simulink model "FOSM"  (R2022b)
settings: Solver=VariableStepAuto  StartTime=0.0  StopTime=10.0  RelTol=1e-3
libraries: fod x2
settings Model: Creator=张倬境  LastModifiedBy=张倬境

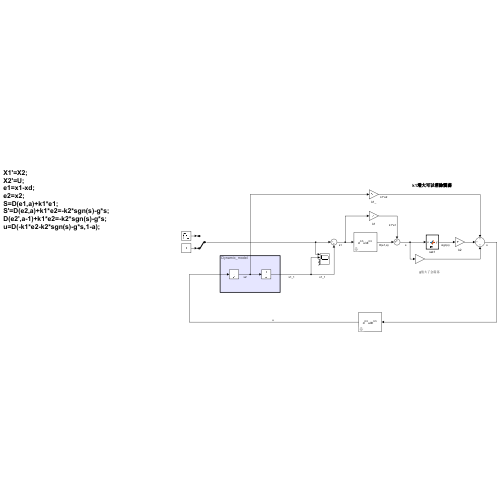
[thumbnail: Simulink's stored preview of the top-level diagram]
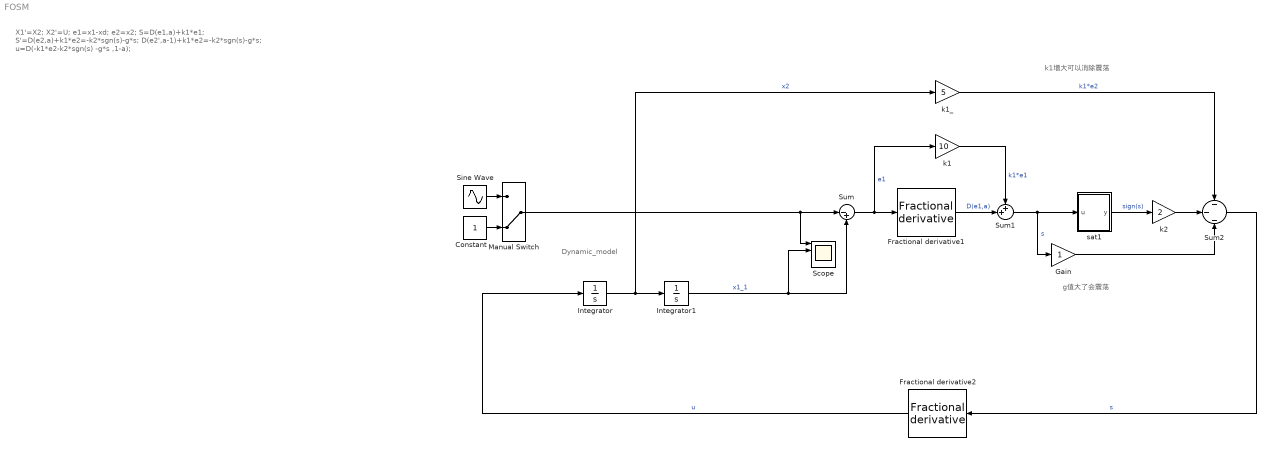
== system FOSM ==
  note: X1'=X2;
      | X2'=U;
      | e1=x1-xd;
      | e2=x2;
      | S=D(e1,a)+k1*e1;
      | S'=D(e2,a)+k1*e2=-k2*sgn(s)-g*s;
      | D(e2',a-1)+k1*e2=-k2*sgn(s)-g*s;
      | u=D(-k1*e2-k2*sgn(s) -g*s ,1-a);
  note: k1增大可以消除震荡
  note: Dynamic_model
  note: g值大了会震荡
  Constant : Constant
  Fractional derivative1 : fod/Fractional derivative  gam=0.5  ww=[0.001; 1000]  n=5  nFod=off
      settings: SourceProductName=FOMCON Toolbox
  Fractional derivative2 : fod/Fractional derivative  gam=0.5  ww=[0.001; 1000]  n=5  nFod=off
      settings: SourceProductName=FOMCON Toolbox
  Gain : Gain
  Integrator : Integrator
  Integrator1 : Integrator
  Manual Switch : ManualSwitch  CurrentSetting=0
  Scope : Scope  NumInputPorts=4
  Sine Wave : Sin  SampleTime=0
  Sum : Sum  Inputs=|-+
  Sum1 : Sum  Inputs=++|
  Sum2 : Sum  Inputs=-|-|-
  k1 : Gain  Gain=10
  k1_ : Gain  Gain=5
  k2 : Gain  Gain=2
  sat1 : MATLAB Function  TreatAsAtomicUnit=on
  wires:
  Sum/1 -> k1/1, Fractional derivative1/1  "e1"
  sat1/1(y) -> k2/1  "sign(s)"
  Gain/1 -> Sum2/3
  Integrator1/1 -> Scope/2, Sum/2  "x1_1"
  Manual Switch/1 -> Scope/1, Sum/1
  k2/1 -> Sum2/2
  Constant/1 -> Manual Switch/2
  k1/1 -> Sum1/1  "k1*e1"
  Fractional derivative1/1 -> Sum1/2  "D(e1,a)"
  Sum1/1 -> Gain/1, sat1/1(u)  "s"
  Fractional derivative2/1 -> Integrator/1  "u"
  k1_/1 -> Sum2/1  "k1*e2"
  Sum2/1 -> Fractional derivative2/1  "s"
  Integrator/1 -> k1_/1, Integrator1/1  "x2"
  Sine Wave/1 -> Manual Switch/1

== matlab function FOSM/sat1 ==
  data: u input; y output
function y = fcn(u)
if(abs(u)>0.01)
    y=sign(u);
else   
    y = 100*u;
end
end
